simulink model "controller_testing"  (R2021a)
settings: Solver=VariableStepAuto  StartTime=0.0  StopTime=10  RelTol=1e-4
values from neighbouring files (symbols this model uses):
  A_hev = [-1/t_P,  0, 0 ... (first row only)    [test.m]
  A_hor = [-1/t_V,  0, 0, 0, 0 ... (first row only)    [test.m]
  A_roll = [-1/t_S, 0; r_S/I_x(1), 0]    [test.m]
  b_hev = [1/t_P; 0; 0]    [test.m]
  b_hor = [1/t_V; 0; 0; 0; 0]    [test.m]
  b_roll = [1/t_S; 0]    [test.m]
  c_alt = [0,0,1,0]    [test.m]
  c_ang = [0,0,1,0]    [test.m]
  c_climb = [0, 1, 0]    [test.m]
  c_rate = [0,1,0]    [test.m]
  c_roll = [0,1]    [test.m]
  c_vel = [0, 0, 0, 0, 1, 0]    [test.m]
undefined symbols (not defined in the file or in its folder): ang_safe, g, T_max, T_max_s, Ts_hev, Ts_hor, Ts_roll, Vec_max
settings Model: Creator=EpEp  LastModifiedBy=EpEp

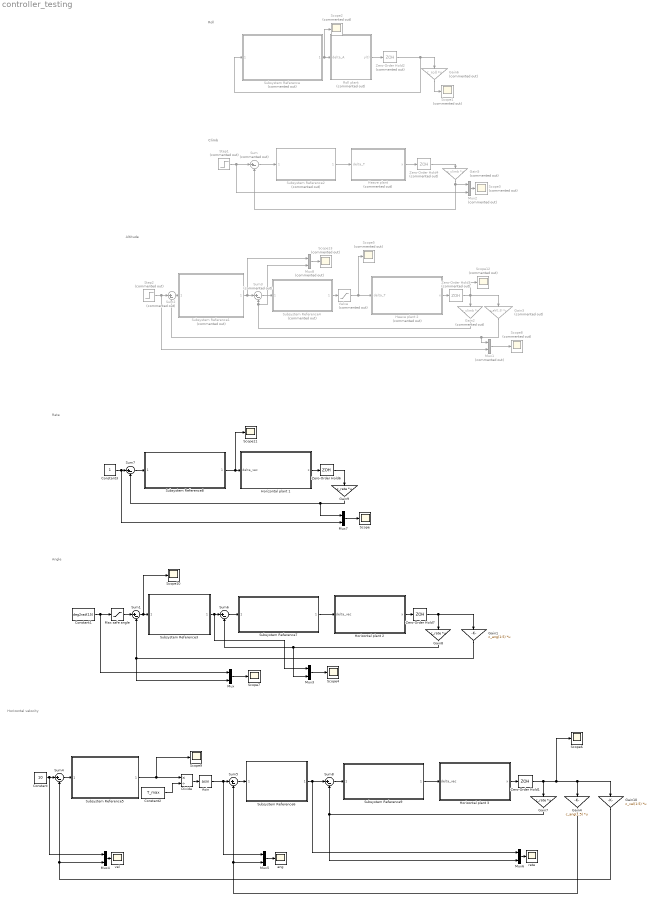
== system controller_testing ==
  note: Horizontal velocity
  note: Angle
  note: Altitude
  note: Climb
  note: Roll
  note: Rate
  Asin : Trigonometry  Operator=asin
  Constant : Constant  Value=10
  Constant1 : Constant  Value=deg2rad(15)
  Constant2 : Constant  Value=T_max
  Constant3 : Constant
  Divide : Product  Inputs=*/
  Gain1 : Gain  Gain=c_ang(1:5)  Multiplication=Matrix(K*u)
  Gain10 : Gain  Gain=c_vel(1:5)  Multiplication=Matrix(K*u)
  Gain2 : Gain  Commented=on  Gain=c_climb  Multiplication=Matrix(K*u)
  Gain3 : Gain  Commented=on  Gain=c_alt(1:3)  Multiplication=Matrix(K*u)
  Gain4 : Gain  Gain=c_ang(1:5)  Multiplication=Matrix(K*u)
  Gain5 : Gain  Commented=on  Gain=c_climb  Multiplication=Matrix(K*u)
  Gain6 : Gain  Commented=on  Gain=c_roll  Multiplication=Matrix(K*u)
  Gain7 : Gain  Gain=c_rate  Multiplication=Matrix(K*u)
  Gain8 : Gain  Gain=c_rate  Multiplication=Matrix(K*u)
  Gain9 : Gain  Gain=c_rate  Multiplication=Matrix(K*u)
  Heave plant : Subsystem  Commented=on
  Heave plant 2 : Subsystem  Commented=on
  Horizontal plant 1 : Subsystem
  Horizontal plant 2 : Subsystem
  Horizontal plant 3 : Subsystem
  Max safe angle : Saturate  UpperLimit=ang_safe  LowerLimit=-ang_safe
  Mux{,3..7} (6 alike) : Mux  Inputs=2
  Mux1 : Mux  Commented=on  Inputs=2
  Mux2 : Mux  Commented=on  Inputs=2
  Mux8 : Mux  Commented=on  Inputs=2
  Roll plant : Subsystem  Commented=on
  Scope{,4,6..7,9..11} (7 alike) : Scope
  Scope{1..3,5,8,12..13} (7 alike) : Scope  Commented=on
  Step1 : Step  Commented=on  Time=50  Before=200  After=-2  SampleTime=0
  Step2 : Step  Commented=on  Time=100  Before=-100  After=0  SampleTime=0
  Subsystem Reference : Subsystem  Commented=on  ReferencedSubsystem=roll_controller
  Subsystem Reference1 : Subsystem  Commented=on  ReferencedSubsystem=alt_control
  Subsystem Reference2 : Subsystem  Commented=on  ReferencedSubsystem=climb_control_PI
  Subsystem Reference3 : Subsystem  ReferencedSubsystem=ang_control
  Subsystem Reference4 : Subsystem  Commented=on  ReferencedSubsystem=climb_control_PI
  Subsystem Reference5 : Subsystem  ReferencedSubsystem=hor_vel_control
  Subsystem Reference6 : Subsystem  ReferencedSubsystem=ang_control
  Subsystem Reference7 : Subsystem  ReferencedSubsystem=rate_controller
  Subsystem Reference8 : Subsystem  ReferencedSubsystem=rate_controller
  Subsystem Reference9 : Subsystem  ReferencedSubsystem=rate_controller
  Sum : Sum  Commented=on  Inputs=|+-
  Sum{1,4..8} (6 alike) : Sum  Inputs=|+-
  Sum2 : Sum  Commented=on  Inputs=|+-
  Sum3 : Sum  Commented=on  Inputs=|+-
  Valve : Saturate  Commented=on  UpperLimit=T_max  LowerLimit=0
  Zero-Order Hold1 : ZeroOrderHold  SampleTime=Ts_hor
  Zero-Order Hold2 : ZeroOrderHold  Commented=on  SampleTime=Ts_roll
  Zero-Order Hold3 : ZeroOrderHold  Commented=on  SampleTime=Ts_hev
  Zero-Order Hold4 : ZeroOrderHold  Commented=on  SampleTime=Ts_hev
  Zero-Order Hold6 : ZeroOrderHold  SampleTime=Ts_hor
  Zero-Order Hold7 : ZeroOrderHold  SampleTime=Ts_hor
  ang : Scope
  rate : Scope
  vel : Scope
  wires:
  Subsystem Reference/1 -> Scope2/1, Roll plant/1(delta_A)
  Roll plant/1(y(t)) -> Zero-Order Hold2/1
  Sum/1 -> Subsystem Reference2/1
  Subsystem Reference2/1 -> Heave plant/1(delta_T)
  Step1/1 -> Mux2/2, Sum/1
  Step2/1 -> Mux1/2, Sum2/1
  Subsystem Reference4/1 -> Valve/1
  Heave plant 2/1(x) -> Zero-Order Hold3/1
  Gain3/1 -> Mux1/1, Sum2/2
  Zero-Order Hold3/1 -> Scope12/1, Gain3/1, Gain2/1
  Sum3/1 -> Subsystem Reference4/1
  Gain2/1 -> Mux8/2, Sum3/2
  Valve/1 -> Scope5/1, Heave plant 2/1(delta_T)
  Sum1/1 -> Scope10/1, Subsystem Reference3/1
  Constant1/1 -> Max safe angle/1, Mux/1
  Mux/1 -> Scope7/1
  Max safe angle/1 -> Sum1/1
  Mux1/1 -> Scope8/1
  Mux2/1 -> Scope3/1
  Gain5/1 -> Sum/2, Mux2/1
  Heave plant/1(x) -> Zero-Order Hold4/1
  Gain6/1 -> Scope1/1
  Zero-Order Hold2/1 -> Subsystem Reference/1, Gain6/1
  Zero-Order Hold4/1 -> Gain5/1
  Subsystem Reference1/1 -> Mux8/1, Sum3/1
  Sum2/1 -> Subsystem Reference1/1
  Sum4/1 -> Subsystem Reference5/1
  Constant/1 -> Mux4/1, Sum4/1
  Horizontal plant 1/1(x) -> Zero-Order Hold6/1
  Zero-Order Hold6/1 -> Gain9/1
  Subsystem Reference8/1 -> Scope11/1, Horizontal plant 1/1(delta_vec)
  Gain9/1 -> Mux7/1, Sum7/2
  Sum7/1 -> Subsystem Reference8/1
  Constant3/1 -> Mux7/2, Sum7/1
  Gain8/1 -> Mux3/2, Sum6/2
  Zero-Order Hold7/1 -> Gain8/1, Gain1/1
  Subsystem Reference7/1 -> Horizontal plant 2/1(delta_vec)
  Horizontal plant 2/1(x) -> Zero-Order Hold7/1
  Sum6/1 -> Subsystem Reference7/1
  Subsystem Reference3/1 -> Mux3/1, Sum6/1
  Gain1/1 -> Mux/2, Sum1/2
  Mux3/1 -> Scope4/1
  Subsystem Reference9/1 -> Horizontal plant 3/1(delta_vec)
  Zero-Order Hold1/1 -> Gain7/1, Scope6/1, Gain10/1, Gain4/1
  Sum8/1 -> Subsystem Reference9/1
  Horizontal plant 3/1(x) -> Zero-Order Hold1/1
  Gain7/1 -> Mux6/2, Sum8/2
  Sum5/1 -> Subsystem Reference6/1
  Gain4/1 -> Sum5/2, Mux5/2
  Gain10/1 -> Sum4/2, Mux4/2
  Mux4/1 -> vel/1
  Mux5/1 -> ang/1
  Mux6/1 -> rate/1
  Subsystem Reference5/1 -> Divide/1, Scope9/1
  Divide/1 -> Asin/1
  Constant2/1 -> Divide/2
  Subsystem Reference6/1 -> Mux6/1, Sum8/1
  Asin/1 -> Mux5/1, Sum5/1
  Mux7/1 -> Scope/1
  Mux8/1 -> Scope13/1

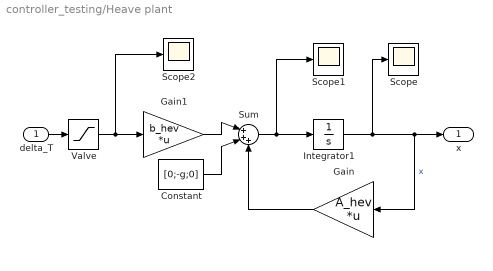
== system controller_testing/Heave plant ==
  delta_T : Inport
  Constant : Constant  Value=[0;-g;0]
  Gain : Gain  Gain=A_hev  Multiplication=Matrix(K*u)
  Gain1 : Gain  Gain=b_hev  Multiplication=Matrix(K*u)
  Integrator1 : Integrator  InitialCondition=[0;0;0]  LimitOutput=on  UpperSaturationLimit=[T_max,inf,0]  LowerSaturationLimit=[0,-inf,-inf]
  Scope : Scope
  Scope1 : Scope
  Scope2 : Scope
  Sum : Sum  Inputs=|+++
  Valve : Saturate  UpperLimit=T_max  LowerLimit=0
  x : Outport
  wires:
  Sum/1 -> Integrator1/1, Scope1/1
  delta_T/1 -> Valve/1
  Gain1/1 -> Sum/1
  Integrator1/1 -> Scope/1, x/1, Gain/1  "x"
  Gain/1 -> Sum/3
  Constant/1 -> Sum/2
  Valve/1 -> Scope2/1, Gain1/1

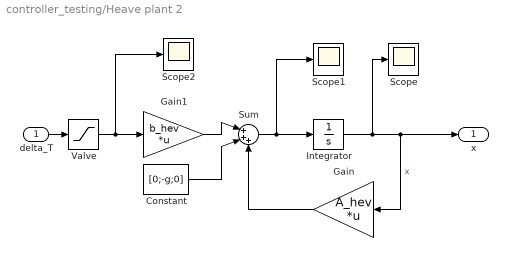
== system controller_testing/Heave plant 2 ==
  delta_T : Inport
  Constant : Constant  Value=[0;-g;0]
  Gain : Gain  Gain=A_hev  Multiplication=Matrix(K*u)
  Gain1 : Gain  Gain=b_hev  Multiplication=Matrix(K*u)
  Integrator : Integrator  InitialCondition=[0;0;0]  LimitOutput=on  UpperSaturationLimit=[T_max,inf,0]  LowerSaturationLimit=[0,-inf,-inf]
  Scope : Scope
  Scope1 : Scope
  Scope2 : Scope
  Sum : Sum  Inputs=|+++
  Valve : Saturate  UpperLimit=T_max  LowerLimit=0
  x : Outport
  wires:
  Sum/1 -> Scope1/1, Integrator/1
  delta_T/1 -> Valve/1
  Gain1/1 -> Sum/1
  Integrator/1 -> Scope/1, x/1, Gain/1  "x"
  Gain/1 -> Sum/3
  Constant/1 -> Sum/2
  Valve/1 -> Scope2/1, Gain1/1

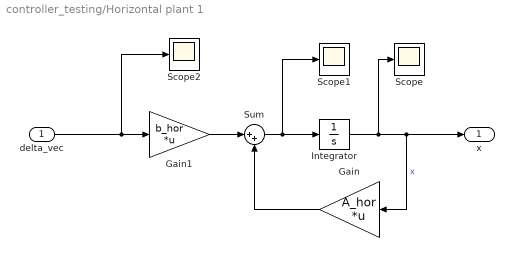
== system controller_testing/Horizontal plant 1 ==
  delta_vec : Inport
  Gain : Gain  Gain=A_hor  Multiplication=Matrix(K*u)
  Gain1 : Gain  Gain=b_hor  Multiplication=Matrix(K*u)
  Integrator : Integrator  InitialCondition=[0;0;0;0;0]  LimitOutput=on  UpperSaturationLimit=[Vec_max,inf,inf,inf,inf]  LowerSaturationLimit=[-Vec_max,-inf,-inf,-inf,-inf]
  Scope : Scope
  Scope1 : Scope
  Scope2 : Scope
  Sum : Sum  Inputs=|++
  x : Outport
  wires:
  Sum/1 -> Integrator/1, Scope1/1
  Gain1/1 -> Sum/1
  Integrator/1 -> Scope/1, x/1, Gain/1  "x"
  Gain/1 -> Sum/2
  delta_vec/1 -> Scope2/1, Gain1/1

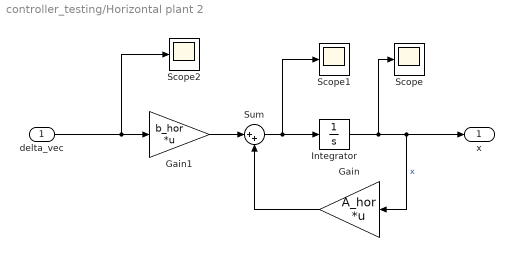
== system controller_testing/Horizontal plant 2 ==
  delta_vec : Inport
  Gain : Gain  Gain=A_hor  Multiplication=Matrix(K*u)
  Gain1 : Gain  Gain=b_hor  Multiplication=Matrix(K*u)
  Integrator : Integrator  InitialCondition=[0;0;0;0;0]  LimitOutput=on  UpperSaturationLimit=[Vec_max,inf,inf,inf,inf]  LowerSaturationLimit=[-Vec_max,-inf,-inf,-inf,-inf]
  Scope : Scope
  Scope1 : Scope
  Scope2 : Scope
  Sum : Sum  Inputs=|++
  x : Outport
  wires:
  Sum/1 -> Integrator/1, Scope1/1
  Gain1/1 -> Sum/1
  Integrator/1 -> Scope/1, x/1, Gain/1  "x"
  Gain/1 -> Sum/2
  delta_vec/1 -> Scope2/1, Gain1/1

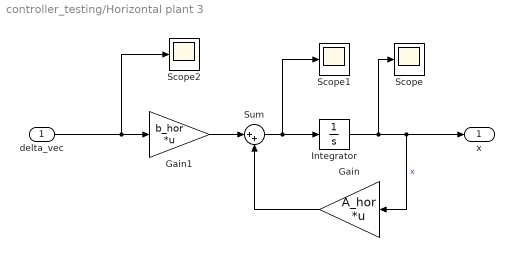
== system controller_testing/Horizontal plant 3 ==
  delta_vec : Inport
  Gain : Gain  Gain=A_hor  Multiplication=Matrix(K*u)
  Gain1 : Gain  Gain=b_hor  Multiplication=Matrix(K*u)
  Integrator : Integrator  InitialCondition=[0;0;0;0;0]  LimitOutput=on  UpperSaturationLimit=[Vec_max,inf,inf,inf,inf]  LowerSaturationLimit=[-Vec_max,-inf,-inf,-inf,-inf]
  Scope : Scope
  Scope1 : Scope
  Scope2 : Scope
  Sum : Sum  Inputs=|++
  x : Outport
  wires:
  Sum/1 -> Integrator/1, Scope1/1
  Gain1/1 -> Sum/1
  Integrator/1 -> Scope/1, x/1, Gain/1  "x"
  Gain/1 -> Sum/2
  delta_vec/1 -> Scope2/1, Gain1/1

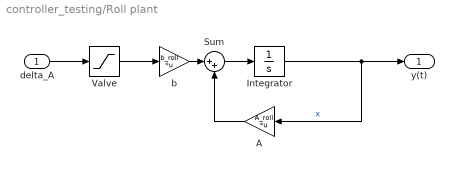
== system controller_testing/Roll plant ==
  delta_A : Inport
  A : Gain  Gain=A_roll  Multiplication=Matrix(K*u)
  Integrator : Integrator  InitialCondition=[0;-1]  LimitOutput=on  UpperSaturationLimit=[1,inf]  LowerSaturationLimit=[-1,-inf]
  Sum : Sum  Inputs=|++
  "Valve " : Saturate  UpperLimit=T_max_s  LowerLimit=-T_max
  b : Gain  Gain=b_roll  Multiplication=Matrix(K*u)
  y(t) : Outport
  wires:
  b/1 -> Sum/1
  A/1 -> Sum/2
  Sum/1 -> Integrator/1
  Integrator/1 -> y(t)/1, A/1  "x"
  "Valve "/1 -> b/1
  delta_A/1 -> "Valve "/1
